simulink model "CF009A_GmOvrlStMgr"  (R2013b)
settings: Solver=FixedStepDiscrete  SolverMode=SingleTasking  StartTime=0.0  StopTime=1  FixedStep=0.002  RelTol=1e-3
values from neighbouring files (symbols this model uses):
  APASTACTV_CNT_U08 = DataDict.Constant    [CF009A_GmOvrlStMgr_DataDict.m]
  APASTCTRLAVL_CNT_U08 = DataDict.Constant    [CF009A_GmOvrlStMgr_DataDict.m]
  ARCHGLBPRM_2MILLISEC_SEC_F32 = DataDict.Constant    [CF009A_GmOvrlStMgr_DataDict.m]
  GmOvrlStMgrApaHwTqThd = DataDict.Calibration    [CF009A_GmOvrlStMgr_DataDict.m]
  GmOvrlStMgrApaHwTqTiThd = DataDict.Calibration    [CF009A_GmOvrlStMgr_DataDict.m]
  GmOvrlStMgrApaMfgEna = DataDict.Calibration    [CF009A_GmOvrlStMgr_DataDict.m]
  GmOvrlStMgrEscMfgEna = DataDict.Calibration    [CF009A_GmOvrlStMgr_DataDict.m]
  GmOvrlStMgrHaptcAmp = DataDict.Calibration    [CF009A_GmOvrlStMgr_DataDict.m]
  GmOvrlStMgrHaptcDurn = DataDict.Calibration    [CF009A_GmOvrlStMgr_DataDict.m]
  GmOvrlStMgrHaptcFrq = DataDict.Calibration    [CF009A_GmOvrlStMgr_DataDict.m]
  GmOvrlStMgrHaptcReactnTi = DataDict.Calibration    [CF009A_GmOvrlStMgr_DataDict.m]
  GmOvrlStMgrHaptcReqTiThd = DataDict.Calibration    [CF009A_GmOvrlStMgr_DataDict.m]
  GmOvrlStMgrHwAgTarLimr = DataDict.Calibration    [CF009A_GmOvrlStMgr_DataDict.m]
  GmOvrlStMgrLkaHwTqThd1 = DataDict.Calibration    [CF009A_GmOvrlStMgr_DataDict.m]
  GmOvrlStMgrLkaHwTqThd2 = DataDict.Calibration    [CF009A_GmOvrlStMgr_DataDict.m]
  GmOvrlStMgrLkaHwTqTiThd1 = DataDict.Calibration    [CF009A_GmOvrlStMgr_DataDict.m]
  GmOvrlStMgrLkaHwTqTiThd2 = DataDict.Calibration    [CF009A_GmOvrlStMgr_DataDict.m]
  GmOvrlStMgrLkaMfgEna = DataDict.Calibration    [CF009A_GmOvrlStMgr_DataDict.m]
  GmOvrlStMgrLoaMtgtnHaptcFbOffTi = DataDict.Calibration    [CF009A_GmOvrlStMgr_DataDict.m]
  GmOvrlStMgrLoaMtgtnHaptcFbOnTi = DataDict.Calibration    [CF009A_GmOvrlStMgr_DataDict.m]
  GmOvrlStMgrLoaMtgtnHaptcFbStrtOnTi = DataDict.Calibration    [CF009A_GmOvrlStMgr_DataDict.m]
  GmOvrlStMgrLoaMtgtnHaptcFbTqMax = DataDict.Calibration    [CF009A_GmOvrlStMgr_DataDict.m]
  GmOvrlStMgrLoaMtgtnHaptcFbTqMin = DataDict.Calibration    [CF009A_GmOvrlStMgr_DataDict.m]
  GmOvrlStMgrLoaMtgtnHaptcFbVehSpdMax = DataDict.Calibration    [CF009A_GmOvrlStMgr_DataDict.m]
  GmOvrlStMgrLoaMtgtnHaptcFbVehSpdMin = DataDict.Calibration    [CF009A_GmOvrlStMgr_DataDict.m]
  GmOvrlStMgrLoaMtgtnHaptcFrq = DataDict.Calibration    [CF009A_GmOvrlStMgr_DataDict.m]
  GmOvrlStMgrLoaMtgtnStrtHaptcAmp = DataDict.Calibration    [CF009A_GmOvrlStMgr_DataDict.m]
  GmOvrlStMgrLoaStIgnCntrThd = DataDict.Calibration    [CF009A_GmOvrlStMgr_DataDict.m]
  GmOvrlStMgrShiftLvrTiThd = DataDict.Calibration    [CF009A_GmOvrlStMgr_DataDict.m]
  GmOvrlStMgrStandStillThd = DataDict.Calibration    [CF009A_GmOvrlStMgr_DataDict.m]
  GmOvrlStMgrStandStillTiThd = DataDict.Calibration    [CF009A_GmOvrlStMgr_DataDict.m]
  HAPTCSTACTV_CNT_U08 = DataDict.Constant    [CF009A_GmOvrlStMgr_DataDict.m]
  HAPTCSTWAIT_CNT_U08 = DataDict.Constant    [CF009A_GmOvrlStMgr_DataDict.m]
  HWOSCNFRQMIN_HZ_F32 = DataDict.Constant    [CF009A_GmOvrlStMgr_DataDict.m]
  LKAFLTCNTRTHD_CNT_U08 = DataDict.Constant    [CF009A_GmOvrlStMgr_DataDict.m]
  LKAFLTTMRTHD_MILLISEC_U32 = DataDict.Constant    [CF009A_GmOvrlStMgr_DataDict.m]
  LKASTPRMNTFAILD_CNT_U08 = DataDict.Constant    [CF009A_GmOvrlStMgr_DataDict.m]
  MILLISECTO100MICROSECCNVN_CNT_U32 = DataDict.Constant    [CF009A_GmOvrlStMgr_DataDict.m]
  NODEBSTEP_CNT_U16 = DataDict.Constant    [CF009A_GmOvrlStMgr_DataDict.m]
undefined symbols (not defined in the file or in its folder): LoaSt1, NtcNr1, NtcSts1, NVM_RequestResultType, SysSt1
libraries: simulink x15, Fil x6, NxtrNvM x4, NxtrLim x4, NxtrAbslt x3, NxtrSign x2, FixdToFloat x1, FloatToFixd x1, LnrIntrpn x1
(part 1 of 8)
Description:
  | Overlay (Position and Torque, Input and Output) State Handler module for GM applications.
  |      This module uses inputs from serial communication (from SER) and from other FDD's to determine the operating state,
  |         which should be received for implementation by an arbiter / limiter function (CF-10 GM Torque Arbitrator).
  |      This function is designed according to the GM LKA SSTS v19.0, LKA System Safety Req'ts V03-07, APA2 SSTS v8, and APA2 System Safety Req'ts EG6 Draft Version.
settings Model: CovMetricSettings=dcmrw  CovFilter=CF09_GMOverlayStateHandler_v002_covfilter  CovHTMLOptions=-sRT=1 -aTS=1 -bRG=1 -bTC=1 -hTR=0 -nFC=0 -scm=1 -bcm=1 -xEv=0  covSaveCumulativeToWorkspaceVar=off  CovSaveSingleToWorkspaceVar=off  CovCumulativeReport=on  Creator=HZ32RQ  LastModifiedBy=TZ5743
settings SolverCC: AutoInsertRateTranBlk=on  InsertRTBMode=Always
settings DataIOCC: LimitDataPoints=off  SaveFormat=Structure  ReturnWorkspaceOutputs=on
settings OptimizationCC: BlockReduction=off  InlineParams=on  ZeroExternalMemoryAtStartup=off  ZeroInternalMemoryAtStartup=off  OptimizeModelRefInitCode=on  LifeSpan=1
settings DebuggingCC: SignalInfNanChecking=error  SignalRangeChecking=warning  UnderspecifiedInitializationDetection=Simplified  SolverPrmCheckMsg=error  InheritedTsInSrcMsg=error  DiscreteInheritContinuousMsg=error  SingleTaskRateTransMsg=error  TasksWithSamePriorityMsg=error  SigSpecEnsureSampleTimeMsg=error  CheckMatrixSingularityMsg=error  ParameterUnderflowMsg=error  ParameterPrecisionLossMsg=error  ParameterTunabilityLossMsg=error  FixptConstUnderflowMsg=warning  FixptConstOverflowMsg=warning  VectorMatrixConversionMsg=error  SignalLabelMismatchMsg=error  UnconnectedInputMsg=error  UnconnectedOutputMsg=error  UnconnectedLineMsg=error  SFcnCompatibilityMsg=error  UniqueDataStoreMsg=warning  BusObjectLabelMismatch=error  RootOutportRequireBusObject=error  AssertControl=DisableAll  ModelReferenceIOMsg=error  ModelReferenceVersionMismatchMessage=warning  ModelReferenceIOMismatchMessage=error  ModelReferenceCSMismatchMessage=warning  ModelReferenceDataLoggingMessage=error  StateNameClashWarn=warning  StrictBusMsg=ErrorOnBusTreatedAsVector  NonBusSignalsTreatedAsBus=error  SFUnexpectedBacktrackingDiag=error  SFInvalidInputDataAccessInChartInitDiag=error  SFNoUnconditionalDefaultTransitionDiag=error  SFTransitionOutsideNaturalParentDiag=error  SFUnconditionalTransitionShadowingDiag=error  SFUndirectedBroadcastEventsDiag=error
settings ModelReferenceCC: ModelReferenceNumInstancesAllowed=Single
settings RTWCC: SystemTargetFile=autosar.tlc  GenCodeOnly=on  TemplateMakefile=ert_default_tmf  Description=AUTOSAR  GenerateReport=on  ProcessScript=autosar_make_rtw_hook  LaunchReport=on
settings CodeAppCC: GenerateComments=off  IgnoreCustomStorageClasses=off  CustomSymbolStrType=$N$R$M  CustomSymbolStrBlkIO=$N$M  SimulinkBlockComments=off
settings STFCustomTargetCC: ParMdlRefBuildCompliant=on  CompOptLevelCompliant=on  IncludeMdlTerminateFcn=off  CombineOutputUpdateFcns=on  SuppressErrorStatus=on  ERTFirstTimeCompliant=on  ERTCustomFileBanners=on  SupportNonFinite=off  SupportComplex=off  SupportContinuousTime=off  SupportNonInlinedSFcns=off  MATLABClassNameForMDSCustomization=Simulink.SoftwareTarget.ERTCustomization  AutosarCompliant=on  GRTInterface=off  SystemTargetFile=autosar.tlc
settings ERTTargetCC: CodeReplacementLibrary=ANSI_C  ConcurrentExecutionCompliant=off  IncludeMdlTerminateFcn=off  SuppressErrorStatus=on  SupportNonFinite=off  SupportComplex=off  ModelStepFunctionPrototypeControlCompliant=off  CPPClassGenCompliant=off  AutosarCompliant=on  InlinedParameterPlacement=NonHierarchical  ERTCustomFileTemplate=example_file_process.tlc  EnableUserReplacementTypes=on

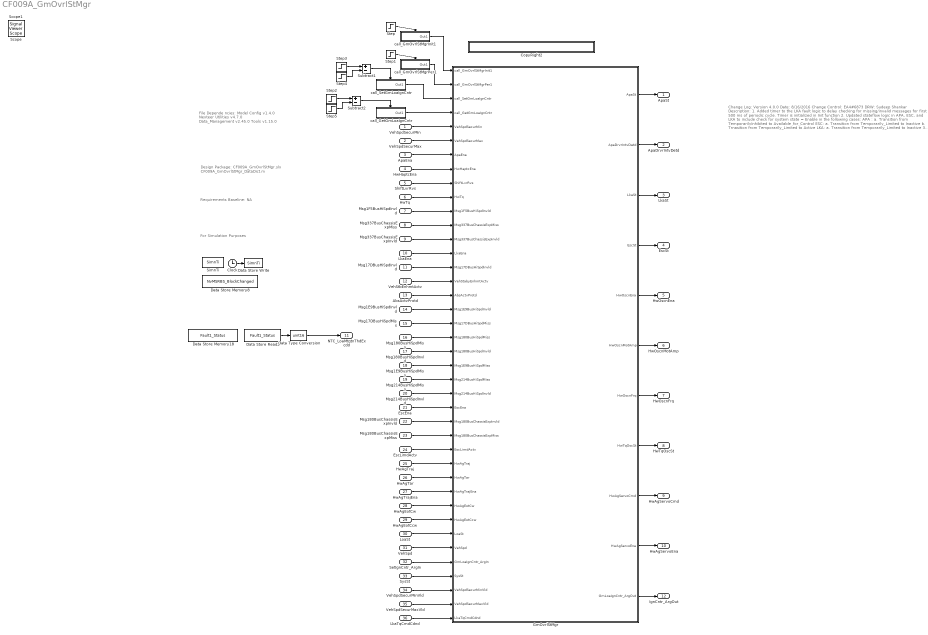
== system CF009A_GmOvrlStMgr ==
  note: File Depende ncies:
      |
      | Model Config v1.4.0
      | Nexteer Utilities v4.7.0
      | Data_Management v2.45.0
      | Tools v1.15.0
  note: Requirements Baseline: NA
  note: Change Log:
      |
      | Version 4.0.0
      | Date: 8/16/2016
      | Change Control: EA4#6873
      | DRW: Sudeep Shankar
      | Description:
      | 1. Added timer to the LKA fault logic to delay checking for missing/invalid messages for first 500 ms of periodic cycle. Timer is initialized in Init function
      | 2. Updated stateflow logic in APA, ESC, and LKA to include check for system state = Enable in the following cases:
      |      APA :
      |     a.  Transition from TemporarilyInhibited to Available_for_Control
      |     ESC:
      |     a. Transition from Temporarily_Limited to Inactive
      |     b. Trnasition from Temporarily_Limited to Active
      |     LKA:
      |     a.  Transition from Temporarily_Limited to Inactive
      |
      | 3. In Stateflow, LoaSt == LoaSt1.LOAST_LIMD check is removed from APA, ESC and LKA based on following requirements update :
      |    CF009A_144, CF009A_160, CF009A_162, CF009A_166, CF009A_169, CF009A_181,  CF009A_191.
      |
      | 4. In Stateflow, following logic is updated in LKA state determination.
      |     a. Transition from Inactive to active condition is changed to:
      |     [LkaEna && (VehSpdSecurMin > GmOvrlStMgrLkaVehSpdLoLim) &&(VehSpdSecurMax < GmOvrlStMgrLkaVehSpdHiLim)]
      |
      |  5. Updated LKA Driver Intervention logic. New input "LkaTqCmdCdnd" is added and sign compared against "HwTq" to help determine if the driver is opposing the LKA command (intervening).
      |     Also, HwTq is now checked against two threshold cals and their corresponding timer elapse condition to determine LKA intervention state.
      |     Timers are initialized in Init function.
      |
      | 6. Removed following calibrations and PIM defintions from Data Dictionary as they are no longer used in design
      |     calibrations:
      | 	a. GmOvrlStMgrLkaHwTqThd
      | 	b. GmOvrlStMgrLkaHwTqTiThd
      |      PIM :
      |      a. LkaFltRefTmr
      |
      | 7. Added folowing new calibrations and PIMdefintions in DD:
      |    calibrations:
      |     a. GmOvrlStMgrLkaHwTqThd1
      |     b. GmOvrlStMgrLkaHwTqThd2
      |     c. GmOvrlStMgrLkaHwTqTiThd1
      |     d. GmOvrlStMgrLkaHwTqTiThd2
      |     PIMs:
      |     a. LkaFltRefTmr1
      |     b. LkaFltRefTmr2
      |
      |
      | Version 3.1.0
      | Date: 6/13/2016
      | Change Control: EA4#5846 & EA4#6268
      | DRW: Price Lefler
      | Description:
      | Model Fixes
      | 	Previously released versions of the FDD referenced requirements links to incorrect Doors modules. These links have been removed from the model and new links need to be
      | 	added to the correct Doors module
      | EA4#5846
      | 	1) Removed LoaStLimdOrSwBasdMtgtn as a PIM and replaced that logic with a temporary variable.
      | 	2) Changed the logic in the HwAgServo subsystem to match the existing source code.
      | 	3) In the Stateflow chart, for all transistions that checked for LoaSt ~= to LOASTNORM_CNT_U08. The logic was changed to instead check for
      | 	    LoaSt == LoaSt1.LOAST_LIMD or LoaSt == LoaSt1.LOAST_SWBASDMTGTN.
      | 	4) In the Stateflow chart, for ESC. The priority for going into Permanently_Failed or Inactive was changed so that going to Permanently_Failed has higher priority.
      | 	5) In the Stateflow chart, for LKA. The condition for going from Inactive to Active was updated to check that VehSpdSecurMin and VehSpdSecrMax are within the LKA vehicle speed limits.
      | 	6) Function Call Generators were updated to match TimeStep properties in the Data Dictionary
      | EA4#6268
      | 	1) For APA, LKA and ESC all transitions to the Temporary Inhibit or Temporarily Limited states now happen when SysSt is equal to SysSt1.SYSST_DI.
      | 	2) Replaced the checks to make sure VehSpdSecurMin and VehSpdSecurMax are within an interval, with VehSpdSecurMinVld and VehSpdSecurMaxVld.
      |
      |
      | V 3.0.0
      | 04/12/2016
      | Change Control #: EA4#9354
      | Author: Ting Zhan
      | Description:
      | -Changed the EngMax to 1.2 for the following cals or consts
      | GmOvrlStMgrHaptcAmp
      | GmOvrlStMgrLoaMtgtnStrtHaptcAmp
      | GmOvrlStMgrLoaMtgtnTqOscnAmpY
      | HWOSCNMOTAMPMAX_MOTNWTMTR_F32
      | -Renamed state HAPTCSTINACTV_CNT_U08 to HAPTCSTINACTVNOTPLS_CNT_U08
      | -Added 2 new states HAPTCSTDI_CNT_U08, HAPTCSTINACTVRDYTOPLS_CNT_U08
      | -Get ref time for PIM "LoaMtgtnHaptcFbStrtOnRefTi" at init
      | -Removed the init value of the Nvm GmLoaIgnCntr in .m file
      |
      |
      | V 2.1.0
      | 02/08/2016
      | Change Control #: EA4#6612
      | Author: Ting Zhan
      | Description:
      | Renamed IgnCntr to GmLoaIgnCntr
      | Renamed runnable to GetGmLoaIgnCntr
      | Renamed runnable to SetGmLoaIgnCntr
      |
      |
      | V 2.0.0
      | 1/29/2016
      | Change Control #: EA4#3628
      | Author: Ting Zhan
      | Description:
      | - Added a HWTorque based intervention for LKA similar to APA implementation.
      | - Added handwheel buzz feature based on number of key cycles in an LoA State of Limited or Software Based Mitigation.
      | - Renamed Outputs from CF009A for SF043A
      | - Added an initial HW Buzz at key on if criteria is met
      |
      |
      | 1/29/2016
      | Change Control #: EA4#2292
      | Author: Ting Zhan
      | Description:
      | - Change input Mfg Enable to Cal
      |
      |
      | 1/11/2016
      | Change Control #: EA4#1886
      | Author: Ting Zhan
      | Description:
      | - Implemented Logic related to elapsed timers in state flow and 'LkaPrmntFlt' determination in model with corresponding PIMs and clients.
      | - Corrected Max value of 'PrevApaIntvRefTi', ‘PrevHaptcReqRefTi’,  ‘PrevShiftLvrRvsRefTi’ and ‘PrevVehStandStillRefTi’
      | - Constant ‘SECTOCNTCNVN_ULS_F32’ name and datatype is not matching. It should be SECTO100MICROSECCNVN_CNT_U32.
      | - In Haptic Inactive ‘Ready_to_Pulse’ state, exit path priorities to be swapped.
      | - In .m file, PIMs ‘HapticActvRefTmr’ and ‘HapticWaitRefTmr’ units should  be ‘Cnt’
      | - Outputs 'HwAgServoCmd', 'HwTqOscAmp' and 'HwTqOscFrq' are not limited
      |
      |
      |
      | V 1.0.0
      | Date: 2Sep2015
      | Change Control #: EA4#
      | Author: Qi Wang
      | Description:
      | - Initial Release Based on EA3 V 1.0.0
      | CR Number: 1600
  note: For Simulation Purposes
  note: Design Package:
      | CF009A_GmOvrlStMgr.slx
      | CF009A_GmOvrlStMgr_DataDict.m
  VehSpdSecurMin : Inport  RequirementInfo={} %GIDa_7bbbe267_ce43_4b60_b622_5d075ab5a072
  VehSpdSecurMax : Inport  RequirementInfo={} %GIDa_fd5f1f1f_cd59_4560_ba05_527fcf9ba805  Port=2
  ApaEna : Inport  RequirementInfo={} %GIDa_58c987c3_a4a9_4e6c_8a4a_a224203eb9dd  Port=3
  HwHaptcEna : Inport  RequirementInfo={} %GIDa_c1836d3e_6741_42ef_bd72_d103282ccab0  Port=4
  ShiftLvrRvs : Inport  RequirementInfo={} %GIDa_9d19d811_5fca_4c7e_8f17_0ac70f07c6a7  Port=5
  HwTq : Inport  RequirementInfo={} %GIDa_00f96092_924a_4c70_b725_19fb4b8cd436  Port=6
  Msg1F5BusHiSpdInvld : Inport  RequirementInfo={} %GIDa_6f2d70cd_1926_4321_9dee_7554482fbf8b  Port=7
  Msg337BusChassisExpMiss : Inport  RequirementInfo={} %GIDa_f5fc5a1e_132d_4584_9efc_717a85058b41  Port=8
  Msg337BusChassisExpInvld : Inport  RequirementInfo={} %GIDa_949ba244_8ccc_4d99_9c77_6ca65b062f1c  Port=9
  LkaEna : Inport  RequirementInfo={} %GIDa_88a05f3b_dfe4_405f_9c8e_7994cd339147  Port=10
  Msg17DBusHiSpdInvld : Inport  RequirementInfo={} %GIDa_8cbe7ea8_62c5_42a7_8a45_c8bd0a389f32  Port=11
  VehStbEnhmtActv : Inport  RequirementInfo={} %GIDa_5d4c55d2_064e_4dff_9b62_bdcf0adeb384  Port=12
  AbsActvProtd : Inport  RequirementInfo={} %GIDa_9bb84497_db14_4e87_b134_1841197e22ad  Port=13
  Msg1E9BusHiSpdInvld : Inport  RequirementInfo={} %GIDa_e5bd1ad0_2b4e_4db5_9cda_d92f9cea83da  Port=14
  Msg17DBusHiSpdMiss : Inport  RequirementInfo={} %GIDa_91061731_a040_4711_9f52_3f28c8043d9f  Port=15
  Msg180BusHiSpdMiss : Inport  RequirementInfo={} %GIDa_e2c55abd_ada3_4ba7_8cf8_e22d5655d2ef  Port=16
  Msg180BusHiSpdInvld : Inport  RequirementInfo={} %GIDa_51e926c6_bade_4e74_9a61_8c131817b0a3  Port=17
  Msg1E9BusHiSpdMiss : Inport  RequirementInfo={} %GIDa_61fccd30_10b4_4c4d_9559_4129c71a97e8  Port=18
  Msg214BusHiSpdMiss : Inport  RequirementInfo={} %GIDa_2256499d_2b4d_4db4_a0f4_a98f6531f54f  Port=19
  Msg214BusHiSpdInvld : Inport  RequirementInfo={} %GIDa_e29b9277_09a6_414b_b6d9_6d18f6a8b946  Port=20
  EscEna : Inport  RequirementInfo={} %GIDa_8deb702d_eace_409f_ba53_d368c7b36238  Port=21
  Msg180BusChassisExpInvld : Inport  RequirementInfo={} %GIDa_35999ec3_357b_45b9_91cc_08edbcf423dc  Port=22
  Msg180BusChassisExpMiss : Inport  RequirementInfo={} %GIDa_ce462fd5_1663_435d_8d07_fc7628c1bc26  Port=23
  EscLimdActv : Inport  RequirementInfo={} %GIDa_a5a4f300_2070_4f47_80b2_1fc7f62c1cb0  Port=24
  HwAgTraj : Inport  RequirementInfo={} %GIDa_79f92fac_b097_411b_8acc_e4e5fbe2f3a0  Port=25
  HwAgTar : Inport  RequirementInfo={} %GIDa_f318b0f5_b20b_4ba5_ae65_bdccd352724a  Port=26
  HwAgTrajEna : Inport  RequirementInfo={} %GIDa_b16c184b_7e5b_452d_94e8_b56e9c4e50b3  Port=27
  HwAgEotCw : Inport  RequirementInfo={} %GIDa_38d90fdb_5098_4dbe_a2fb_d0dc697a3f47  Port=28
  HwAgEotCcw : Inport  RequirementInfo={} %GIDa_5439553e_af05_4303_a56c_782ccd5e07bf  Port=29
  LoaSt : Inport  RequirementInfo={} %GIDa_ac300c63_fbe5_4c77_8194_80c5c0abb310  Port=30
  VehSpd : Inport  RequirementInfo={} %GIDa_0655883f_361f_4b25_8846_5f02e07a817e  Port=31
  SetIgnCntr_ArgIn : Inport  RequirementInfo={} %GIDa_222ce18f_26d3_4980_86f9_d766e4416ef3  Port=32
  SysSt : Inport  RequirementInfo={} %GIDa_c4f2ffde_f272_4ee9_a9b0_f91698b0fddb  Port=33
  VehSpdSecurMinVld : Inport  RequirementInfo={} %GIDa_88e7639d_20df_4183_81af_b12264c5eb7c  Port=34
  VehSpdSecurMaxVld : Inport  RequirementInfo={} %GIDa_b2c9a74c_a850_4107_b5d6_6fcc7f1788f4  Port=35
  LkaTqCmdCdnd : Inport  RequirementInfo={} %GIDa_0bf1ebc6_bbc5_43b5_8902_9ea7b321e13b  Port=36
  Clock : Clock
  CopyRight2 : Subsystem  Description=|  mask(Copyright Information){none=on}
      | Copyright info block.                                               
      |                                                                     
      | Place copyright information at the top of every subsystem in design.
      mask prompts: none "No parameters"
      mask help: Place copyright information at the top of every subsystem in design.
      mask Display:
      | NxtrConf = 'Nexteer Confidential';
      | 
      | sys = bdroot; %handle for the current model ("system")
      | first = get_param(sys,'Created');
      | if(isempty(first))
      |     first = datestr(now,'yyyy');
      | else
      |     first = first(end-3:end);  %year is last four digits
      | end
      | 
      | last = get_param(sys,'LastModifiedDate');
      | if isempty(last)
      |     last = datestr(now,'yyyy');
      | else
      |     last = last(end-3:end);
      | end
      | 
      | if strcmp(first,last)
      |     fprintf('%s -- Copyright %s Nexteer',NxtrConf,first)
      | else
      |     fprintf('%s -- %s%s- %s Nexteer',NxtrConf,char(169),first,last)
      | end
  Data Store Memory18 : DataStoreMemory  DataStoreName=Fault1_Status  InitialValue=NtcSts1.NTCSTS_PASSD  OutDataTypeStr=Enum: NtcSts1
  Data Store Memory8 : DataStoreMemory  DataStoreName=NvMSRBS_BlockChanged
  Data Store Read2 : DataStoreRead  DataStoreName=Fault1_Status  SampleTime=.004
  Data Store Write : DataStoreWrite  DataStoreName=SimnTi
  Data Type Conversion : DataTypeConversion  OutDataTypeStr=uint16
  GmOvrlStMgr : Subsystem
  SimnTi : DataStoreMemory  DataStoreName=SimnTi
  Step : Step  Time=.001  Before=1  After=0  SampleTime=0
  Step1 : Step  Time=0.002  SampleTime=0
  Step2 : Step  Time=9.7  SampleTime=0.002
  Step3 : Step  Time=6.7  SampleTime=0.002
  Step4 : Step  Time=6.701  SampleTime=0.002
  Step5 : Step  Time=9.701  SampleTime=0.002
  Subtract1 : Sum  Inputs=+-
  Subtract2 : Sum  Inputs=+-
  call_GetGmLoaIgnCntr : Subsystem  TreatAsAtomicUnit=on
  call_GmOvrlStMgrInit1 : Subsystem  TreatAsAtomicUnit=on
  call_GmOvrlStMgrPer1 : Subsystem  TreatAsAtomicUnit=on
  call_SetGmLoaIgnCntr : Subsystem  TreatAsAtomicUnit=on
  ApaSt : Outport  RequirementInfo={} %GIDa_1da87020_2114_47f8_bd6a_dcf122c70ef9
  ApaDrvrIntvDetd : Outport  RequirementInfo={} %GIDa_48488018_a40b_476d_93d8_71a8e5b9b9ef  Port=2
  LkaSt : Outport  RequirementInfo={} %GIDa_aa71e542_5f04_4ff7_aa01_7ea85d72a732  Port=3
  EscSt : Outport  RequirementInfo={} %GIDa_6ce0db0a_f918_4040_a381_a66b37fb6372  Port=4
  HwOscnEna : Outport  RequirementInfo={} %GIDa_d1eaba6b_7fd6_4e51_9c42_dd5776a9d81a  Port=5
  HwOscnMotAmp : Outport  RequirementInfo={} %GIDa_6478e093_5f0f_4e63_b8a8_e013203d7b8e  Port=6
  HwOscnFrq : Outport  RequirementInfo={} %GIDa_504b29d3_d93e_4132_9764_2035c150d4e2  Port=7
  HwTqOscSt : Outport  RequirementInfo={} %GIDa_2b10f20f_5f69_4141_8c42_1f825b03cbb6  Port=8
  HwAgServoCmd : Outport  RequirementInfo={} %GIDa_9f759655_0441_4e00_a886_f2396882726e  Port=9
  HwAgServoEna : Outport  RequirementInfo={} %GIDa_b7cb585f_686e_4513_927a_8f385b666f58  Port=10
  NTC_LoaMtgtnThdExcdd : Outport  Port=11
  IgnCntr_ArgOut : Outport  RequirementInfo={} %GIDa_ad6b84c6_e8ae_499c_aeb7_ca01ae52e293  Port=12
  Scope : SignalViewerScope  IOType=viewer  RefreshTime=0.035000
  Scope1 : SignalViewerScope  IOType=viewer  RefreshTime=0.035000
  wires:
  Step/1 -> call_GmOvrlStMgrInit1/Enable
  call_GmOvrlStMgrInit1/1(Out1) -> GmOvrlStMgr/1(call_GmOvrlStMgrInit1)
  Clock/1 -> Data Store Write/1
  HwAgEotCcw/1 -> GmOvrlStMgr/33(HwAgEotCcw)
  Msg17DBusHiSpdMiss/1 -> GmOvrlStMgr/19(Msg17DBusHiSpdMiss)
  Msg214BusHiSpdMiss/1 -> GmOvrlStMgr/23(Msg214BusHiSpdMiss)
  VehStbEnhmtActv/1 -> GmOvrlStMgr/16(VehStabyEnhmtActv)
  LoaSt/1 -> GmOvrlStMgr/34(LoaSt)
  Msg180BusChassisExpInvld/1 -> GmOvrlStMgr/26(Msg180BusChassisExpInvld)
  EscEna/1 -> GmOvrlStMgr/25(EscEna)
  Msg214BusHiSpdInvld/1 -> GmOvrlStMgr/24(Msg214BusHiSpdInvld)
  EscLimdActv/1 -> GmOvrlStMgr/28(EscLimdActv)
  Msg1E9BusHiSpdInvld/1 -> GmOvrlStMgr/18(Msg1E9BusHiSpdInvld)
  HwAgEotCw/1 -> GmOvrlStMgr/32(HwAgEotCw)
  HwAgTar/1 -> GmOvrlStMgr/30(HwAgTar)
  Msg180BusHiSpdInvld/1 -> GmOvrlStMgr/21(Msg180BusHiSpdInvld)
  Msg180BusChassisExpMiss/1 -> GmOvrlStMgr/27(Msg180BusChassisExpMiss)
  HwAgTraj/1 -> GmOvrlStMgr/29(HwAgTraj)
  HwAgTrajEna/1 -> GmOvrlStMgr/31(HwAgTrajEna)
  Msg1E9BusHiSpdMiss/1 -> GmOvrlStMgr/22(Msg1E9BusHiSpdMiss)
  AbsActvProtd/1 -> GmOvrlStMgr/17(AbsActvProtd)
  Msg180BusHiSpdMiss/1 -> GmOvrlStMgr/20(Msg180BusHiSpdMiss)
  ShiftLvrRvs/1 -> GmOvrlStMgr/9(ShiftLvrRvs)
  HwHaptcEna/1 -> GmOvrlStMgr/8(HwHaptcEna)
  VehSpdSecurMin/1 -> GmOvrlStMgr/5(VehSpdSecurMin)
  HwTq/1 -> GmOvrlStMgr/10(HwTq)
  ApaEna/1 -> GmOvrlStMgr/7(ApaEna)
  VehSpdSecurMax/1 -> GmOvrlStMgr/6(VehSpdSecurMax)
  Msg337BusChassisExpMiss/1 -> GmOvrlStMgr/12(Msg337BusChassisExpMiss)
  LkaEna/1 -> GmOvrlStMgr/14(LkaEna)
  Msg337BusChassisExpInvld/1 -> GmOvrlStMgr/13(Msg337BusChassisExpInvld)
  Msg1F5BusHiSpdInvld/1 -> GmOvrlStMgr/11(Msg1F5BusHiSpdInvld)
  Msg17DBusHiSpdInvld/1 -> GmOvrlStMgr/15(Msg17DBusHiSpdInvld)
  GmOvrlStMgr/3(LkaSt) -> LkaSt/1
  GmOvrlStMgr/1(ApaSt) -> ApaSt/1
  GmOvrlStMgr/7(HwOscnFrq) -> HwOscnFrq/1
  GmOvrlStMgr/2(ApaDrvrIntvDetd) -> ApaDrvrIntvDetd/1
  GmOvrlStMgr/5(HwOscnEna) -> HwOscnEna/1
  GmOvrlStMgr/4(EscSt) -> EscSt/1
  GmOvrlStMgr/8(HwTqOscSt) -> HwTqOscSt/1
  GmOvrlStMgr/10(HwAgServoEna) -> HwAgServoEna/1
  GmOvrlStMgr/6(HwOscnMotAmp) -> HwOscnMotAmp/1
  GmOvrlStMgr/9(HwAgServoCmd) -> HwAgServoCmd/1
  VehSpd/1 -> GmOvrlStMgr/35(VehSpd)
  Step1/1 -> call_GmOvrlStMgrPer1/Enable
  call_GmOvrlStMgrPer1/1(Out1) -> GmOvrlStMgr/2(call_GmOvrlStMgrPer1)
  Data Store Read2/1 -> Data Type Conversion/1
  Data Type Conversion/1 -> NTC_LoaMtgtnThdExcdd/1
  Subtract1/1 -> call_SetGmLoaIgnCntr/Enable
  Step3/1 -> Subtract1/1
  Step4/1 -> Subtract1/2
  call_SetGmLoaIgnCntr/1(Out1) -> GmOvrlStMgr/3(call_SetGmLoaIgnCntr)
  GmOvrlStMgr/11(GmLoaIgnCntr_ArgOut) -> IgnCntr_ArgOut/1
  call_GetGmLoaIgnCntr/1(Out1) -> GmOvrlStMgr/4(call_GetGmLoaIgnCntr)
  Subtract2/1 -> call_GetGmLoaIgnCntr/Enable
  Step2/1 -> Subtract2/1
  Step5/1 -> Subtract2/2
  SetIgnCntr_ArgIn/1 -> GmOvrlStMgr/36(GmLoaIgnCntr_ArgIn)
  SysSt/1 -> GmOvrlStMgr/37(SysSt)
  VehSpdSecurMinVld/1 -> GmOvrlStMgr/38(VehSpdSecurMinVld)
  VehSpdSecurMaxVld/1 -> GmOvrlStMgr/39(VehSpdSecurMaxVld)
  LkaTqCmdCdnd/1 -> GmOvrlStMgr/40(LkaTqCmdCdnd)

== system CF009A_GmOvrlStMgr/CopyRight2 ==

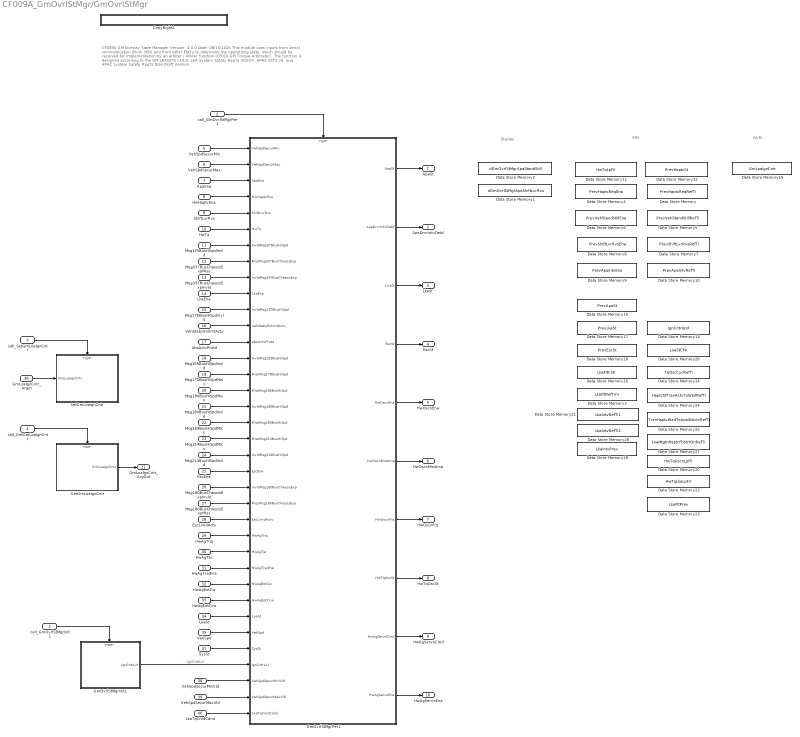
== system CF009A_GmOvrlStMgr/GmOvrlStMgr ==
  note: Display
  note: PIM
  note: CF009A GM Overlay State Manager
      | Version: 4.0.0      Date: 08/16/2016
      |
      | This module uses inputs from serial communication (from SER) and from other FDD's to determine the operationg state, which should be received for
      |  implementation by an arbiter / limiter function (CF010 GM Torque Arbitrator).
      | The function is designed according to the GM LKASSTS v19.0, LKA System Safety Req'ts V03-07, APA2 SSTS v8, and APA2 System Safety Req'ts
      | EG6 Draft Version.
  note: NVM
  call_GmOvrlStMgrInit1 : Inport  RequirementInfo={} %GIDa_bfdeb5c8_34d3_4847_8322_14533b8a1ec7
  call_GmOvrlStMgrPer1 : Inport  RequirementInfo={} %GIDa_f1c70cb1_f5af_488b_94e7_678758a8a022  Port=2
  call_SetGmLoaIgnCntr : Inport  RequirementInfo={} %GIDa_ff2bfb54_15ff_4807_b9c1_1ae04284f107  Port=3
  call_GetGmLoaIgnCntr : Inport  RequirementInfo={} %GIDa_d9e077ff_6eeb_4f29_bb2a_14860485513b  Port=4
  VehSpdSecurMin : Inport  RequirementInfo={} %GIDa_b8091ed2_b107_43da_94c8_c56552fc988c  Port=5
  VehSpdSecurMax : Inport  RequirementInfo={} %GIDa_59971eb5_90c5_49de_a4c1_590931baa8e9  Port=6
  ApaEna : Inport  RequirementInfo={} %GIDa_630d0546_94a0_490c_bab9_431cefe95881  Port=7
  HwHaptcEna : Inport  RequirementInfo={} %GIDa_31ffdbe0_9b4e_4bb5_a1af_0dfec7e6ec0e  Port=8
  ShiftLvrRvs : Inport  RequirementInfo={} %GIDa_63174388_6f70_4886_b3e9_35d6ec40a8f5  Port=9
  HwTq : Inport  RequirementInfo={} %GIDa_a99ee987_d404_43a8_87dc_37acf15e08f1  Port=10
  Msg1F5BusHiSpdInvld : Inport  RequirementInfo={} %GIDa_5b03c7bf_07da_47c1_9319_c99374b26ba6  Port=11
  Msg337BusChassisExpMiss : Inport  RequirementInfo={} %GIDa_0801239f_e708_4e40_9e1a_65ee040f82af  Port=12
  Msg337BusChassisExpInvld : Inport  RequirementInfo={} %GIDa_5e25a3e6_0d79_4249_84d2_25ff211d6a11  Port=13
  LkaEna : Inport  RequirementInfo={} %GIDa_ee314012_a633_4edf_92e7_fd7e5d68c42c  Port=14
  Msg17DBusHiSpdInvld : Inport  RequirementInfo={} %GIDa_db4437e0_d90f_41dd_9531_42692e56a100  Port=15
  VehStabyEnhmtActv : Inport  RequirementInfo={} %GIDa_41d6bf18_4c0d_4f1a_bf51_e9d5f5e795f4  Port=16
  AbsActvProtd : Inport  RequirementInfo={} %GIDa_b59a68d2_7b30_4aad_9c24_69e0f640c144  Port=17
  Msg1E9BusHiSpdInvld : Inport  RequirementInfo={} %GIDa_c57732b2_a067_4023_97f7_34a74984b5d9  Port=18
  Msg17DBusHiSpdMiss : Inport  RequirementInfo={} %GIDa_5cafc9e2_1e89_4de5_a869_fd73bfc6f214  Port=19
  Msg180BusHiSpdMiss : Inport  RequirementInfo={} %GIDa_461ee87b_770c_4110_bae5_4842bcb9a860  Port=20
  Msg180BusHiSpdInvld : Inport  RequirementInfo={} %GIDa_f6207d6b_82ea_466e_b4a0_cf1b696f6c4f  Port=21
  Msg1E9BusHiSpdMiss : Inport  RequirementInfo={} %GIDa_7ad493df_fa5d_42ed_9d38_192ebf40e8b5  Port=22
  Msg214BusHiSpdMiss : Inport  RequirementInfo={} %GIDa_1d1aeb69_55a4_40cc_a862_76dc2e1f1a51  Port=23
  Msg214BusHiSpdInvld : Inport  RequirementInfo={} %GIDa_c6498202_a587_49e0_be56_6d49c5cb272f  Port=24
  EscEna : Inport  RequirementInfo={} %GIDa_62a13558_b222_4e20_a70e_f5d3a94fd09d  Port=25
  Msg180BusChassisExpInvld : Inport  RequirementInfo={} %GIDa_e8a68cf5_18ae_4c29_8cc4_2d1270e129ef  Port=26
  Msg180BusChassisExpMiss : Inport  RequirementInfo={} %GIDa_cffc153b_feb7_4622_b4c7_8565efcc8405  Port=27
  EscLimdActv : Inport  RequirementInfo={} %GIDa_d2894f3d_00ed_46f1_a7e0_cb9f46029934  Port=28
  HwAgTraj : Inport  RequirementInfo={} %GIDa_a5cccee1_ac77_4988_ae20_20dcbc55879e  Port=29
  HwAgTar : Inport  RequirementInfo={} %GIDa_2070ca93_c137_43b9_a399_80ce0b48b5eb  Port=30
  HwAgTrajEna : Inport  RequirementInfo={} %GIDa_429f2cda_e11d_48ea_a2eb_5fd27ea07d5d  Port=31
  HwAgEotCw : Inport  RequirementInfo={} %GIDa_ad668d17_35ff_44df_9860_75efaa7dcff5  Port=32
  HwAgEotCcw : Inport  RequirementInfo={} %GIDa_6fcb7483_eba6_49fd_8c2d_44cfcdfa3c4c  Port=33
  LoaSt : Inport  RequirementInfo={} %GIDa_c65d3410_035d_4077_bc84_ccb160e747ee  Port=34
  VehSpd : Inport  RequirementInfo={} %GIDa_c856a574_7f16_48bc_8e9f_ce028307095c  Port=35
  GmLoaIgnCntr_ArgIn : Inport  RequirementInfo={} %GIDa_17debced_ceaa_4286_9660_12ab83092e72  Port=36
  SysSt : Inport  RequirementInfo={} %GIDa_db6698cc_5478_4e2d_847d_9b6602c7c745  Port=37
  VehSpdSecurMinVld : Inport  RequirementInfo={} %GIDa_4236d746_d610_433f_8f69_14f2e50f3e01  Port=38
  VehSpdSecurMaxVld : Inport  RequirementInfo={} %GIDa_17244990_ef13_42d9_a209_197127a40d0b  Port=39
  LkaTqCmdCdnd : Inport  RequirementInfo={} %GIDa_f684c441_1ccd_4fe5_89b3_b25c84d0e4f3  Port=40
  CopyRight2 : Subsystem  Description=|  mask(Copyright Information){none=on}
      | Copyright info block.                                               
      |                                                                     
      | Place copyright information at the top of every subsystem in design.
      mask prompts: none "No parameters"
      mask help: Place copyright information at the top of every subsystem in design.
      mask Display:
      | NxtrConf = 'Nexteer Confidential';
      | 
      | sys = bdroot; %handle for the current model ("system")
      | first = get_param(sys,'Created');
      | if(isempty(first))
      |     first = datestr(now,'yyyy');
      | else
      |     first = first(end-3:end);  %year is last four digits
      | end
      | 
      | last = get_param(sys,'LastModifiedDate');
      | if isempty(last)
      |     last = datestr(now,'yyyy');
      | else
      |     last = last(end-3:end);
      | end
      | 
      | if strcmp(first,last)
      |     fprintf('%s -- Copyright %s Nexteer',NxtrConf,first)
      | else
      |     fprintf('%s -- %s%s- %s Nexteer',NxtrConf,char(169),first,last)
      | end
  Data Store Memory : DataStoreMemory  DataStoreName=PrevHaptcReqRefTi  StateMustResolveToSignalObject=on
  Data Store Memory1 : DataStoreMemory  DataStoreName=dGmOvrlStMgrApaShiftLvrRvs  ReadBeforeWriteMsg=warning  WriteAfterWriteMsg=warning  WriteAfterReadMsg=warning  StateMustResolveToSignalObject=on
  Data Store Memory10 : DataStoreMemory  DataStoreName=PrevApaIntvRefTi  StateMustResolveToSignalObject=on
  Data Store Memory11 : DataStoreMemory  DataStoreName=HwTqLpFil  InitialValue=[]  OutDataTypeStr=Bus: FilLpRec1  StateMustResolveToSignalObject=on
  Data Store Memory12 : DataStoreMemory  DataStoreName=PrevHaptcSt  StateMustResolveToSignalObject=on
  Data Store Memory13 : DataStoreMemory  DataStoreName=IgnCntrUpd  StateMustResolveToSignalObject=on
  Data Store Memory14 : DataStoreMemory  DataStoreName=TqOscCycRefTi  StateMustResolveToSignalObject=on
  Data Store Memory15 : DataStoreMemory  DataStoreName=PrevApaSt  StateMustResolveToSignalObject=on
  Data Store Memory16 : DataStoreMemory  DataStoreName=LkaFltCntr  StateMustResolveToSignalObject=on
  Data Store Memory17 : DataStoreMemory  DataStoreName=PrevLkaSt  StateMustResolveToSignalObject=on
  Data Store Memory18 : DataStoreMemory  DataStoreName=PrevEscSt  StateMustResolveToSignalObject=on
  Data Store Memory19 : DataStoreMemory  DataStoreName=GmLoaIgnCntr  StateMustResolveToSignalObject=on
  Data Store Memory2 : DataStoreMemory  DataStoreName=dGmOvrlStMgrApaStandStill  ReadBeforeWriteMsg=warning  WriteAfterWriteMsg=warning  WriteAfterReadMsg=warning  StateMustResolveToSignalObject=on
  Data Store Memory20 : DataStoreMemory  DataStoreName=HwTqOscnLpFil  InitialValue=[]  OutDataTypeStr=Bus: FilLpRec1  StateMustResolveToSignalObject=on
  Data Store Memory21 : DataStoreMemory  DataStoreName=LkaIntvRefTi1  StateMustResolveToSignalObject=on
  Data Store Memory22 : DataStoreMemory  DataStoreName=HwTqLkaLpFil  InitialValue=[]  OutDataTypeStr=Bus: FilLpRec1  StateMustResolveToSignalObject=on
  Data Store Memory23 : DataStoreMemory  DataStoreName=LkaFltPrev  StateMustResolveToSignalObject=on
  Data Store Memory24 : DataStoreMemory  DataStoreName=HaptcStTranActvToWaitRefTi  StateMustResolveToSignalObject=on
  Data Store Memory25 : DataStoreMemory  DataStoreName=TranHaptcWaitToApaStActvRefTi  StateMustResolveToSignalObject=on
  Data Store Memory26 : DataStoreMemory  DataStoreName=LoaStChk  StateMustResolveToSignalObject=on
  Data Store Memory27 : DataStoreMemory  DataStoreName=LoaMtgtnHaptcFbStrtOnRefTi  StateMustResolveToSignalObject=on
  Data Store Memory28 : DataStoreMemory  DataStoreName=LkaIntvRefTi2  StateMustResolveToSignalObject=on
  Data Store Memory29 : DataStoreMemory  DataStoreName=LkaIntvPrev  StateMustResolveToSignalObject=on
  Data Store Memory3 : DataStoreMemory  DataStoreName=LkaFltRefTmr  StateMustResolveToSignalObject=on
  Data Store Memory4 : DataStoreMemory  DataStoreName=PrevHaptcReqEna  StateMustResolveToSignalObject=on
  Data Store Memory5 : DataStoreMemory  DataStoreName=PrevVehStandStillRefTi  StateMustResolveToSignalObject=on
  Data Store Memory6 : DataStoreMemory  DataStoreName=PrevVehStandStillEna  StateMustResolveToSignalObject=on
  Data Store Memory7 : DataStoreMemory  DataStoreName=PrevShiftLvrRvsRefTi  StateMustResolveToSignalObject=on
  Data Store Memory8 : DataStoreMemory  DataStoreName=PrevShiftLvrRvsEna  StateMustResolveToSignalObject=on
  Data Store Memory9 : DataStoreMemory  DataStoreName=PrevApaIntvEna  StateMustResolveToSignalObject=on
  GetGmLoaIgnCntr : Subsystem  TreatAsAtomicUnit=on
  GmOvrlStMgrInit1 : Subsystem
  GmOvrlStMgrPer1 : Subsystem
  SetGmLoaIgnCntr : Subsystem  TreatAsAtomicUnit=on
  ApaSt : Outport  RequirementInfo={} %GIDa_193ab0a0_dd30_4f7a_a182_b40d65e68801
  ApaDrvrIntvDetd : Outport  RequirementInfo={} %GIDa_95f09734_cbc3_4313_97fb_8e7ce07b83e7  Port=2
  LkaSt : Outport  RequirementInfo={} %GIDa_f59e91f0_fe76_4f29_916e_753e2c200ee2  Port=3
  EscSt : Outport  RequirementInfo={} %GIDa_2ee994e2_76da_417c_9ecc_5cdaff7fdb07  Port=4
  HwOscnEna : Outport  RequirementInfo={} %GIDa_b07bcc61_0d4b_46ce_858f_1ec9923a4410  Port=5
  HwOscnMotAmp : Outport  RequirementInfo={} %GIDa_383f6d57_11d9_4c9c_96d5_280289cf0bf4  Port=6
  HwOscnFrq : Outport  RequirementInfo={} %GIDa_eb40bf25_ad1a_4bfa_84f8_c35cfbbb6e89  Port=7
  HwTqOscSt : Outport  RequirementInfo={} %GIDa_bc5f2e70_87e0_4721_81db_1e3b10ef5210  Port=8
  HwAgServoCmd : Outport  RequirementInfo={} %GIDa_d6fe4083_7b94_42ce_a480_0d60d9985d01  Port=9
  HwAgServoEna : Outport  RequirementInfo={} %GIDa_722b84bb_e5ce_45c4_8c9a_727e36bd79d4  Port=10
  GmLoaIgnCntr_ArgOut : Outport  RequirementInfo={} %GIDa_7560ed43_c5ad_460b_9c89_fb0a39bbc3de  Port=11
  wires:
  VehSpdSecurMin/1 -> GmOvrlStMgrPer1/1(VehSpdSecurMin)
  VehSpdSecurMax/1 -> GmOvrlStMgrPer1/2(VehSpdSecurMax)
  ApaEna/1 -> GmOvrlStMgrPer1/3(ApaEna)
  HwHaptcEna/1 -> GmOvrlStMgrPer1/4(HwHaptcEna)
  ShiftLvrRvs/1 -> GmOvrlStMgrPer1/5(ShiftLvrRvs)
  HwTq/1 -> GmOvrlStMgrPer1/6(HwTq)
  Msg1F5BusHiSpdInvld/1 -> GmOvrlStMgrPer1/7(InvldMsg1F5BusHiSpd)
  LkaEna/1 -> GmOvrlStMgrPer1/10(LkaEna)
  Msg17DBusHiSpdInvld/1 -> GmOvrlStMgrPer1/11(InvldMsg17DBusHiSpd)
  EscEna/1 -> GmOvrlStMgrPer1/21(EscEna)
  EscLimdActv/1 -> GmOvrlStMgrPer1/24(EscLimdActv)
  HwAgTraj/1 -> GmOvrlStMgrPer1/25(HwAgTraj)
  HwAgTar/1 -> GmOvrlStMgrPer1/26(HwAgTar)
  HwAgTrajEna/1 -> GmOvrlStMgrPer1/27(HwAgTrajEna)
  HwAgEotCw/1 -> GmOvrlStMgrPer1/28(HwAgEotCw)
  HwAgEotCcw/1 -> GmOvrlStMgrPer1/29(HwAgEotCcw)
  LoaSt/1 -> GmOvrlStMgrPer1/30(LoaSt)
  GmOvrlStMgrPer1/1(ApaSt) -> ApaSt/1
  GmOvrlStMgrPer1/2(ApaDrvrIntvDetd) -> ApaDrvrIntvDetd/1
  GmOvrlStMgrPer1/3(LkaSt) -> LkaSt/1
  GmOvrlStMgrPer1/4(EscSt) -> EscSt/1
  GmOvrlStMgrPer1/5(HwOscnEna) -> HwOscnEna/1
  GmOvrlStMgrPer1/6(HwOscnMotAmp) -> HwOscnMotAmp/1
  GmOvrlStMgrPer1/7(HwOscnFrq) -> HwOscnFrq/1
  GmOvrlStMgrPer1/8(HwTqOscSt) -> HwTqOscSt/1
  GmOvrlStMgrPer1/9(HwAgServoCmd) -> HwAgServoCmd/1
  GmOvrlStMgrPer1/10(HwAgServoEna) -> HwAgServoEna/1
  call_GmOvrlStMgrPer1/1 -> GmOvrlStMgrPer1/Trigger
  call_GmOvrlStMgrInit1/1 -> GmOvrlStMgrInit1/Trigger
  Msg17DBusHiSpdMiss/1 -> GmOvrlStMgrPer1/15(MissMsg17DBusHiSpd)
  Msg180BusHiSpdMiss/1 -> GmOvrlStMgrPer1/16(MissMsg180BusHiSpd)
  Msg180BusHiSpdInvld/1 -> GmOvrlStMgrPer1/17(InvldMsg180BusHiSpd)
  Msg1E9BusHiSpdMiss/1 -> GmOvrlStMgrPer1/18(MissMsg1E9BusHiSpd)
  Msg214BusHiSpdMiss/1 -> GmOvrlStMgrPer1/19(MissMsg214BusHiSpd)
  Msg214BusHiSpdInvld/1 -> GmOvrlStMgrPer1/20(InvldMsg214BusHiSpd)
  AbsActvProtd/1 -> GmOvrlStMgrPer1/13(AbsActvProtd)
  VehStabyEnhmtActv/1 -> GmOvrlStMgrPer1/12(VehStabyEnhmtActv)
  Msg1E9BusHiSpdInvld/1 -> GmOvrlStMgrPer1/14(InvldMsg1E9BusHiSpd)
  Msg337BusChassisExpMiss/1 -> GmOvrlStMgrPer1/8(MissMsg337BusChassisExp)
  Msg337BusChassisExpInvld/1 -> GmOvrlStMgrPer1/9(InvldMsg337BusChassisExp)
  Msg180BusChassisExpInvld/1 -> GmOvrlStMgrPer1/22(InvldMsg180BusChassisExp)
  Msg180BusChassisExpMiss/1 -> GmOvrlStMgrPer1/23(MissMsg180BusChassisExp)
  VehSpd/1 -> GmOvrlStMgrPer1/31(VehSpd)
  call_SetGmLoaIgnCntr/1 -> SetGmLoaIgnCntr/Trigger
  call_GetGmLoaIgnCntr/1 -> GetGmLoaIgnCntr/Trigger
  GetGmLoaIgnCntr/1(GmLoaIgnCntr) -> GmLoaIgnCntr_ArgOut/1
  GmLoaIgnCntr_ArgIn/1 -> SetGmLoaIgnCntr/1(GmLoaIgnCntr)
  SysSt/1 -> GmOvrlStMgrPer1/32(SysSt)
  GmOvrlStMgrInit1/1(IgnCntrLcl) -> GmOvrlStMgrPer1/33(IgnCntrLcl)  "IgnCntrLcl"
  VehSpdSecurMaxVld/1 -> GmOvrlStMgrPer1/35(VehSpdSecurMaxVld)
  VehSpdSecurMinVld/1 -> GmOvrlStMgrPer1/34(VehSpdSecurMinVld)
  LkaTqCmdCdnd/1 -> GmOvrlStMgrPer1/36("LkaTqCmdCdnd ")

== system CF009A_GmOvrlStMgr/call_GetGmLoaIgnCntr ==
  Enable : EnablePort
  CopyRight1 : Subsystem  Description=|  mask(Copyright Information){none=on}
      | Copyright info block.                                               
      |                                                                     
      | Place copyright information at the top of every subsystem in design.
      mask prompts: none "No parameters"
      mask help: Place copyright information at the top of every subsystem in design.
      mask Display:
      | NxtrConf = 'Nexteer Confidential';
      | 
      | sys = bdroot; %handle for the current model ("system")
      | first = get_param(sys,'Created');
      | if(isempty(first))
      |     first = datestr(now,'yyyy');
      | else
      |     first = first(end-3:end);  %year is last four digits
      | end
      | 
      | last = get_param(sys,'LastModifiedDate');
      | if isempty(last)
      |     last = datestr(now,'yyyy');
      | else
      |     last = last(end-3:end);
      | end
      | 
      | if strcmp(first,last)
      |     fprintf('%s -- Copyright %s Nexteer',NxtrConf,first)
      | else
      |     fprintf('%s -- %s%s- %s Nexteer',NxtrConf,char(169),first,last)
      | end
  FunctionCallGenerator : simulink/Ports & Subsystems/Function-Call Generator  sample_time=0.002  numberOfIterations=1
  Out1 : Outport
  wires:
  FunctionCallGenerator/1 -> Out1/1

== system CF009A_GmOvrlStMgr/call_GmOvrlStMgrInit1 ==
  Enable : EnablePort
  CopyRight2 : Subsystem  Description=|  mask(Copyright Information){none=on}
      | Copyright info block.                                               
      |                                                                     
      | Place copyright information at the top of every subsystem in design.
      mask prompts: none "No parameters"
      mask help: Place copyright information at the top of every subsystem in design.
      mask Display:
      | NxtrConf = 'Nexteer Confidential';
      | 
      | sys = bdroot; %handle for the current model ("system")
      | first = get_param(sys,'Created');
      | if(isempty(first))
      |     first = datestr(now,'yyyy');
      | else
      |     first = first(end-3:end);  %year is last four digits
      | end
      | 
      | last = get_param(sys,'LastModifiedDate');
      | if isempty(last)
      |     last = datestr(now,'yyyy');
      | else
      |     last = last(end-3:end);
      | end
      | 
      | if strcmp(first,last)
      |     fprintf('%s -- Copyright %s Nexteer',NxtrConf,first)
      | else
      |     fprintf('%s -- %s%s- %s Nexteer',NxtrConf,char(169),first,last)
      | end
  FunctionCallGenerator : simulink/Ports & Subsystems/Function-Call Generator  sample_time=0.002  numberOfIterations=1
  Out1 : Outport
  wires:
  FunctionCallGenerator/1 -> Out1/1

== system CF009A_GmOvrlStMgr/call_GmOvrlStMgrPer1 ==
  Enable : EnablePort
  CopyRight2 : Subsystem  Description=|  mask(Copyright Information){none=on}
      | Copyright info block.                                               
      |                                                                     
      | Place copyright information at the top of every subsystem in design.
      mask prompts: none "No parameters"
      mask help: Place copyright information at the top of every subsystem in design.
      mask Display:
      | NxtrConf = 'Nexteer Confidential';
      | 
      | sys = bdroot; %handle for the current model ("system")
      | first = get_param(sys,'Created');
      | if(isempty(first))
      |     first = datestr(now,'yyyy');
      | else
      |     first = first(end-3:end);  %year is last four digits
      | end
      | 
      | last = get_param(sys,'LastModifiedDate');
      | if isempty(last)
      |     last = datestr(now,'yyyy');
      | else
      |     last = last(end-3:end);
      | end
      | 
      | if strcmp(first,last)
      |     fprintf('%s -- Copyright %s Nexteer',NxtrConf,first)
      | else
      |     fprintf('%s -- %s%s- %s Nexteer',NxtrConf,char(169),first,last)
      | end
  FunctionCallGenerator : simulink/Ports & Subsystems/Function-Call Generator  sample_time=0.002  numberOfIterations=1
  Out1 : Outport
  wires:
  FunctionCallGenerator/1 -> Out1/1

== system CF009A_GmOvrlStMgr/call_SetGmLoaIgnCntr ==
  Enable : EnablePort
  CopyRight1 : Subsystem  Description=|  mask(Copyright Information){none=on}
      | Copyright info block.                                               
      |                                                                     
      | Place copyright information at the top of every subsystem in design.
      mask prompts: none "No parameters"
      mask help: Place copyright information at the top of every subsystem in design.
      mask Display:
      | NxtrConf = 'Nexteer Confidential';
      | 
      | sys = bdroot; %handle for the current model ("system")
      | first = get_param(sys,'Created');
      | if(isempty(first))
      |     first = datestr(now,'yyyy');
      | else
      |     first = first(end-3:end);  %year is last four digits
      | end
      | 
      | last = get_param(sys,'LastModifiedDate');
      | if isempty(last)
      |     last = datestr(now,'yyyy');
      | else
      |     last = last(end-3:end);
      | end
      | 
      | if strcmp(first,last)
      |     fprintf('%s -- Copyright %s Nexteer',NxtrConf,first)
      | else
      |     fprintf('%s -- %s%s- %s Nexteer',NxtrConf,char(169),first,last)
      | end
  FunctionCallGenerator : simulink/Ports & Subsystems/Function-Call Generator  sample_time=0.002  numberOfIterations=1
  Out1 : Outport
  wires:
  FunctionCallGenerator/1 -> Out1/1

== system CF009A_GmOvrlStMgr/GmOvrlStMgr/CopyRight2 ==

== system CF009A_GmOvrlStMgr/GmOvrlStMgr/GetGmLoaIgnCntr ==
  function : TriggerPort  TriggerType=function-call
  CopyRight2 : Subsystem  Description=|  mask(Copyright Information){none=on}
      | Copyright info block.                                               
      |                                                                     
      | Place copyright information at the top of every subsystem in design.
      mask prompts: none "No parameters"
      mask help: Place copyright information at the top of every subsystem in design.
      mask Display:
      | NxtrConf = 'Nexteer Confidential';
      | 
      | sys = bdroot; %handle for the current model ("system")
      | first = get_param(sys,'Created');
      | if(isempty(first))
      |     first = datestr(now,'yyyy');
      | else
      |     first = first(end-3:end);  %year is last four digits
      | end
      | 
      | last = get_param(sys,'LastModifiedDate');
      | if isempty(last)
      |     last = datestr(now,'yyyy');
      | else
      |     last = last(end-3:end);
      | end
      | 
      | if strcmp(first,last)
      |     fprintf('%s -- Copyright %s Nexteer',NxtrConf,first)
      | else
      |     fprintf('%s -- %s%s- %s Nexteer',NxtrConf,char(169),first,last)
      | end
  Data Store Read2 : DataStoreRead  DataStoreName=GmLoaIgnCntr
  GmLoaIgnCntr : Outport  RequirementInfo={} %GIDa_8783a1e7_bf83_4e54_8c7f_69afe613aa85
  wires:
  Data Store Read2/1 -> GmLoaIgnCntr/1

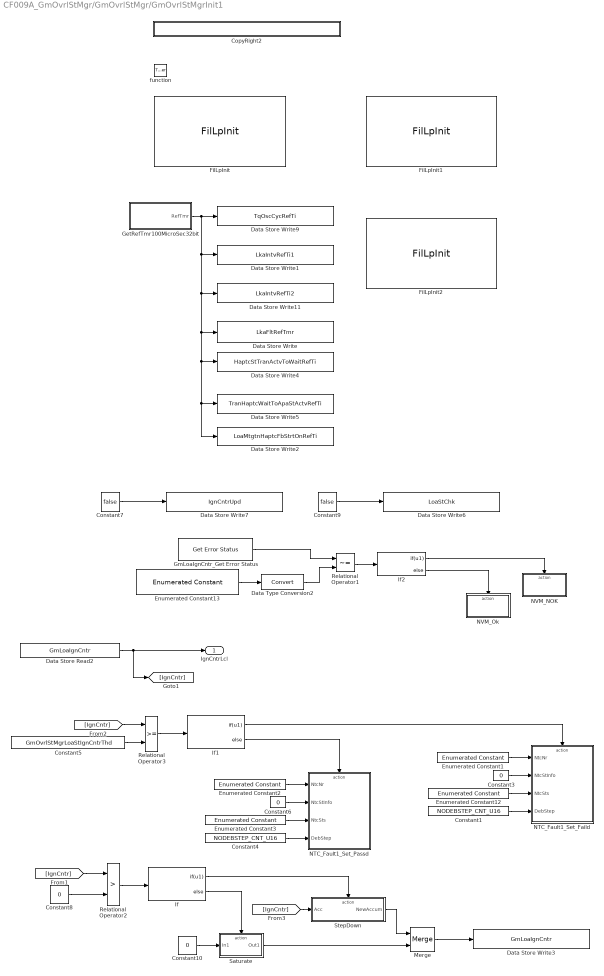
== system CF009A_GmOvrlStMgr/GmOvrlStMgr/GmOvrlStMgrInit1 ==
  function : TriggerPort  TriggerType=function-call
  Constant1 : Constant  Value=NODEBSTEP_CNT_U16
  Constant10 : Constant  Value=0  OutDataTypeStr=Inherit: Inherit via back propagation
  Constant3 : Constant  Value=0
  Constant4 : Constant  Value=NODEBSTEP_CNT_U16
  Constant5 : Constant  Value=GmOvrlStMgrLoaStIgnCntrThd
  Constant6 : Constant  Value=0
  Constant7 : Constant  Value=false  OutDataTypeStr=boolean
      settings: AttributesFormatString=%<OutDataTypeStr>
  Constant8 : Constant  Value=0  OutDataTypeStr=Inherit: Inherit via back propagation
  Constant9 : Constant  Value=false  OutDataTypeStr=boolean
      settings: AttributesFormatString=%<OutDataTypeStr>
  CopyRight2 : Subsystem  Description=|  mask(Copyright Information){none=on}
      | Copyright info block.                                               
      |                                                                     
      | Place copyright information at the top of every subsystem in design.
      mask prompts: none "No parameters"
      mask help: Place copyright information at the top of every subsystem in design.
      mask Display:
      | NxtrConf = 'Nexteer Confidential';
      | 
      | sys = bdroot; %handle for the current model ("system")
      | first = get_param(sys,'Created');
      | if(isempty(first))
      |     first = datestr(now,'yyyy');
      | else
      |     first = first(end-3:end);  %year is last four digits
      | end
      | 
      | last = get_param(sys,'LastModifiedDate');
      | if isempty(last)
      |     last = datestr(now,'yyyy');
      | else
      |     last = last(end-3:end);
      | end
      | 
      | if strcmp(first,last)
      |     fprintf('%s -- Copyright %s Nexteer',NxtrConf,first)
      | else
      |     fprintf('%s -- %s%s- %s Nexteer',NxtrConf,char(169),first,last)
      | end
  Data Store Read2 : DataStoreRead  DataStoreName=GmLoaIgnCntr
  Data Store Write : DataStoreWrite  DataStoreName=LkaFltRefTmr
  Data Store Write1 : DataStoreWrite  DataStoreName=LkaIntvRefTi1
  Data Store Write11 : DataStoreWrite  DataStoreName=LkaIntvRefTi2
  Data Store Write2 : DataStoreWrite  DataStoreName=LoaMtgtnHaptcFbStrtOnRefTi
  Data Store Write3 : DataStoreWrite  DataStoreName=GmLoaIgnCntr
  Data Store Write4 : DataStoreWrite  DataStoreName=HaptcStTranActvToWaitRefTi
  Data Store Write5 : DataStoreWrite  DataStoreName=TranHaptcWaitToApaStActvRefTi
  Data Store Write6 : DataStoreWrite  DataStoreName=LoaStChk
  Data Store Write7 : DataStoreWrite  DataStoreName=IgnCntrUpd
  Data Store Write9 : DataStoreWrite  DataStoreName=TqOscCycRefTi
  Data Type Conversion2 : DataTypeConversion
  Enumerated Constant1 : simulink/Sources/Enumerated Constant  OutDataTypeStr=Enum: NtcNr1  Value=NtcNr1.NTCNR_0X0E2  SampleTime=inf
  Enumerated Constant12 : simulink/Sources/Enumerated Constant  OutDataTypeStr=Enum: NtcSts1  Value=NtcSts1.NTCSTS_FAILD  SampleTime=inf
  Enumerated Constant2 : simulink/Sources/Enumerated Constant  OutDataTypeStr=Enum: NtcNr1  Value=NtcNr1.NTCNR_0X0E2  SampleTime=inf
  Enumerated Constant3 : simulink/Sources/Enumerated Constant  OutDataTypeStr=Enum: NtcSts1  Value=NtcSts1.NTCSTS_PASSD  SampleTime=inf
  Enumerated Constant13 : simulink/Sources/Enumerated Constant  RequirementInfo={} %GIDa_ee669472_e14f_4de1_96fa_884e99ea1b0f  OutDataTypeStr=Enum: NVM_RequestResultType  Value=NVM_RequestResultType.NVM_REQ_OK  SampleTime=inf
  FilLpInit : Fil/FilLpInit  Ic=0  Ts=ARCHGLBPRM_2MILLISEC_SEC_F32  Freq=GmOvrlStMgrApaHwTqFilFrq  StVar=HwTqLpFil
  FilLpInit1 : Fil/FilLpInit  RequirementInfo={} %GIDa_124ca31b_d283_403c_a039_8e21522c33e0  Ic=0  Ts=ARCHGLBPRM_2MILLISEC_SEC_F32  Freq=GmOvrlStMgrHwTqFilFrq  StVar=HwTqOscnLpFil
  FilLpInit2 : Fil/FilLpInit  RequirementInfo={} %GIDa_ef6b43f8_e898_4716_8eee_949de5d28bcd  Ic=0  Ts=ARCHGLBPRM_2MILLISEC_SEC_F32  Freq=GmOvrlStMgrLkaHwTqFilFrq  StVar=HwTqLkaLpFil
  GetRefTmr100MicroSec32bit : Subsystem
  GmLoaIgnCntr_Get Error Status : NxtrNvM/Get Error Status  FuncName=Get Error Status  NvMBlockName=GmLoaIgnCntr  VoidFuncRtn=on  ReqResPtr_DSN=NvMGES_ReqResPtr  Return_DSN=NvMGES_ReqResPtr
      settings: AttributesFormatString=%<FuncName>
  If : If  IfExpression=u1
  If1 : If  IfExpression=u1
  If2 : If  IfExpression=u1
  Merge : Merge
  NTC_Fault1_Set_Faild : Subsystem  mask(SetNTC){}
      mask help: SetNTC library block
  NTC_Fault1_Set_Passd : Subsystem  mask(SetNTC){}
      mask help: SetNTC library block
  NVM_NOK : Subsystem  RequirementInfo={} %GIDa_af0ee7bf_3c15_4274_9edd_eaaa701d55a2  TreatAsAtomicUnit=on
  NVM_Ok : Subsystem  RequirementInfo={} %GIDa_f86a2880_cd6c_4bdb_b9fc_57f2701c9ba2  TreatAsAtomicUnit=on
  Relational Operator1 : RelationalOperator  Operator=~=  OutDataTypeStr=boolean
  Relational Operator2 : RelationalOperator  Priority=1  Operator=>  OutDataTypeStr=boolean
      settings: AttributesFormatString=%<Priority>
  Relational Operator3 : RelationalOperator  Priority=0  OutDataTypeStr=boolean
      settings: AttributesFormatString=%<Priority>
  Saturate : Subsystem  TreatAsAtomicUnit=on
  StepDown : Subsystem  TreatAsAtomicUnit=on
  IgnCntrLcl : Outport  RequirementInfo={} %GIDa_a2181d5b_976f_4227_86d8_42c569d8ec74
  wires:
  Constant7/1 -> Data Store Write7/1
  Relational Operator1/1 -> If2/1
  If2/1 -> NVM_NOK/Action
  Data Store Read2/1 -> IgnCntrLcl/1, [IgnCntr]
  If2/2 -> NVM_Ok/Action
  GmLoaIgnCntr_Get Error Status/1 -> Relational Operator1/1
  Enumerated Constant13/1 -> Data Type Conversion2/1
  Data Type Conversion2/1 -> Relational Operator1/2
  Merge/1 -> Data Store Write3/1
  Saturate/1(Out1) -> Merge/2
  StepDown/1(NewAccum) -> Merge/1
  Constant10/1 -> Saturate/1(In1)
  If/2 -> Saturate/Action
  If/1 -> StepDown/Action
  [IgnCntr] -> Relational Operator2/1
  Constant8/1 -> Relational Operator2/2
  Relational Operator2/1 -> If/1
  If1/2 -> NTC_Fault1_Set_Passd/Action
  If1/1 -> NTC_Fault1_Set_Faild/Action
  [IgnCntr] -> Relational Operator3/1
  Constant5/1 -> Relational Operator3/2
  Relational Operator3/1 -> If1/1
  Enumerated Constant1/1 -> NTC_Fault1_Set_Faild/1(NtcNr)
  Enumerated Constant12/1 -> NTC_Fault1_Set_Faild/3(NtcSts)
  Constant1/1 -> NTC_Fault1_Set_Faild/4(DebStep)
  Constant3/1 -> NTC_Fault1_Set_Faild/2(NtcStInfo)
  Enumerated Constant2/1 -> NTC_Fault1_Set_Passd/1(NtcNr)
  Enumerated Constant3/1 -> NTC_Fault1_Set_Passd/3(NtcSts)
  Constant4/1 -> NTC_Fault1_Set_Passd/4(DebStep)
  Constant6/1 -> NTC_Fault1_Set_Passd/2(NtcStInfo)
  Constant9/1 -> Data Store Write6/1
  [IgnCntr] -> StepDown/1(Acc)
  GetRefTmr100MicroSec32bit/1(RefTmr) -> Data Store Write11/1, Data Store Write/1, Data Store Write5/1, Data Store Write2/1, Data Store Write4/1, Data Store Write1/1, Data Store Write9/1
